simulink model "PI"  (R2024a)
settings: Solver=VariableStepAuto  StartTime=0.0  StopTime=5  RelTol=1e-3
values from neighbouring files (symbols this model uses):
  B = 0    [Parameters.m]
  J = 0.006    [Parameters.m]
  Ls = 0.4    [Parameters.m]
  p = 4    [Parameters.m]
  Rs = 0.02    [Parameters.m]
  samplingTime = 50    [Parameters.m]
  Sm = 0.2205    [Parameters.m]
libraries: slpidlib x3, spsTriangleGeneratorLib x1
settings Model: Creator=anugr  LastModifiedBy=anugr
settings DataIOCC: ReturnWorkspaceOutputs=off

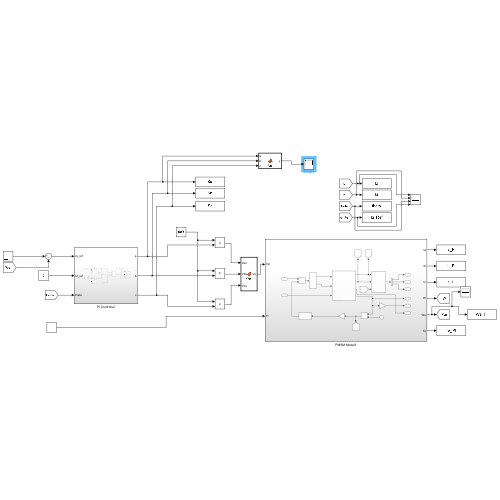
[thumbnail: Simulink's stored preview of the top-level diagram]
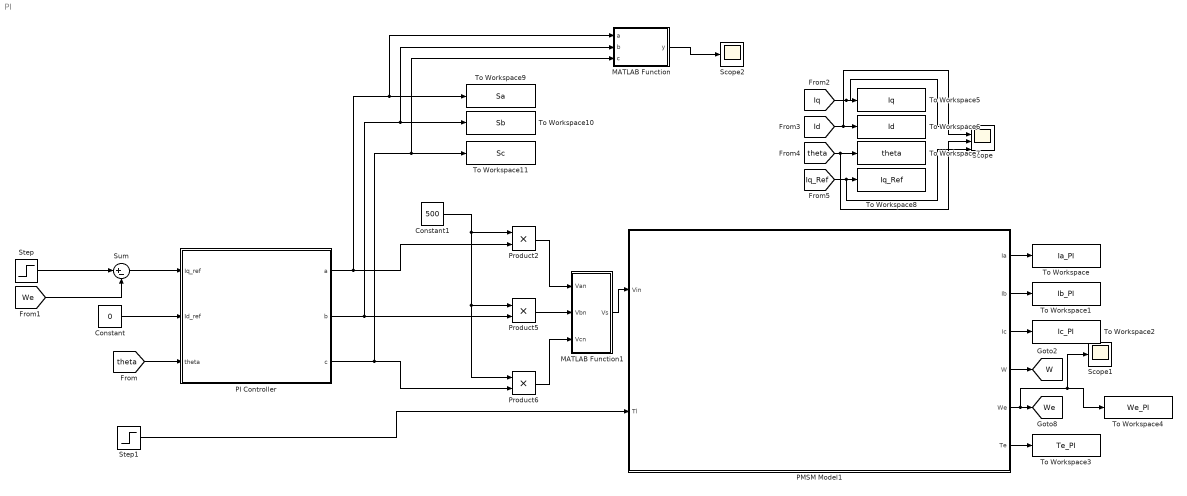
== system PI ==
  Constant : Constant  Value=0
  Constant1 : Constant  Value=500
  MATLAB Function : MATLAB Function  TreatAsAtomicUnit=on
  MATLAB Function1 : MATLAB Function  TreatAsAtomicUnit=on
  PI Controller : Subsystem
  PMSM Model1 : Subsystem
  Product2 : Product
  Product5 : Product
  Product6 : Product
  Scope : Scope  NumInputPorts=4
  Scope1 : Scope
  Scope2 : Scope
  Step : Step  Time=2.5  Before=200  After=400  SampleTime=0
  Step1 : Step  Time=2.5  After=0  SampleTime=0
  Sum : Sum  Inputs=|+-
  To Workspace : ToWorkspace  VariableName=Ia_PI  SaveFormat=Timeseries  SampleTime=-1
  To Workspace1 : ToWorkspace  VariableName=Ib_PI  SaveFormat=Timeseries  SampleTime=-1
  To Workspace10 : ToWorkspace  VariableName=Sb  SampleTime=samplingTime*1e-5
  To Workspace11 : ToWorkspace  VariableName=Sc  SampleTime=samplingTime*1e-5
  To Workspace2 : ToWorkspace  VariableName=Ic_PI  SaveFormat=Timeseries  SampleTime=-1
  To Workspace3 : ToWorkspace  VariableName=Te_PI  SaveFormat=Timeseries  SampleTime=-1
  To Workspace4 : ToWorkspace  VariableName=We_PI  SampleTime=samplingTime * 1e-5
  To Workspace5 : ToWorkspace  VariableName=Iq  SampleTime=samplingTime*1e-5
  To Workspace6 : ToWorkspace  VariableName=Id  SampleTime=samplingTime*1e-5
  To Workspace7 : ToWorkspace  VariableName=theta  SampleTime=samplingTime*1e-5
  To Workspace8 : ToWorkspace  VariableName=Iq_Ref  SampleTime=samplingTime*1e-5
  To Workspace9 : ToWorkspace  VariableName=Sa  SampleTime=samplingTime*1e-5
  tag scope: W=global, We=global
  wires:
  Step/1 -> Sum/1
  Sum/1 -> PI Controller/1(Iq_ref)
  Constant/1 -> PI Controller/2(Id_ref)
  MATLAB Function1/1(Vs) -> PMSM Model1/1(Vin)
  Product5/1 -> MATLAB Function1/2(Vbn)
  PI Controller/1(a) -> MATLAB Function/1(a), To Workspace9/1, Product2/2
  PI Controller/3(c) -> MATLAB Function/3(c), To Workspace11/1, Product6/2
  Constant1/1 -> Product5/1, Product6/1, Product2/1
  PI Controller/2(b) -> MATLAB Function/2(b), To Workspace10/1, Product5/2
  Product6/1 -> MATLAB Function1/3(Vcn)
  Product2/1 -> MATLAB Function1/1(Van)
  PMSM Model1/3(Ic) -> To Workspace2/1
  PMSM Model1/1(Ia) -> To Workspace/1
  PMSM Model1/2(Ib) -> To Workspace1/1
  PMSM Model1/4(W) -> [W]
  PMSM Model1/5(We) -> Scope1/1, To Workspace4/1, [We]
  PMSM Model1/6(Te) -> To Workspace3/1
  Step1/1 -> PMSM Model1/2(Tl)
  [theta] -> PI Controller/3(theta)
  [We] -> Sum/2
  [Iq] -> Scope/1, To Workspace5/1
  [Id] -> Scope/2, To Workspace6/1
  [theta] -> Scope/3, To Workspace7/1
  [Iq_Ref] -> Scope/4, To Workspace8/1
  MATLAB Function/1(y) -> Scope2/1

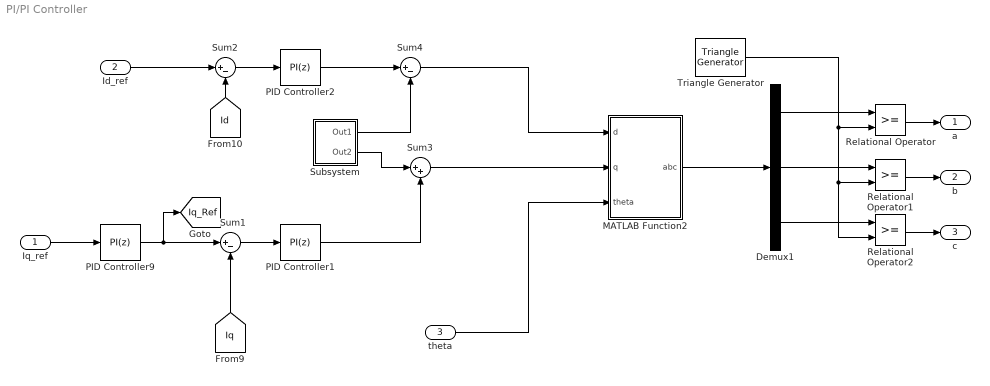
== system PI/PI Controller ==
  Iq_ref : Inport
  Id_ref : Inport  Port=2
  theta : Inport  Port=3
  Demux1 : Demux  Outputs=3
  MATLAB Function2 : MATLAB Function  TreatAsAtomicUnit=on
  PID Controller1 : slpidlib/PID Controller  Controller=PI  Form=Parallel  TimeDomain=Discrete-time  UseExternalTs=off  SampleTime=-1  IntegratorMethod=Forward Euler  FilterMethod=Forward Euler  ControllerParametersSource=internal  P=100  I=30  UseKiTs=off  D=0  UseExternalDerivativeSource=off  N=100  UseFilter=on  TunerSelectOption=Transfer Function Based (PID Tuner App)  InitialConditionSource=internal  InitialConditionForIntegrator=0  InitialConditionForFilter=0  DifferentiatorICPrevScaledInput=0  ExternalReset=none  TrackingMode=off  Kt=1  LimitOutput=off  SatLimitsSource=internal  UpperSaturationLimit=inf  LowerSaturationLimit=-inf  LinearizeAsGain=on  AntiWindupMode=none  Kb=1  LimitIntegrator=off  UpperIntegratorSaturationLimit=inf  LowerIntegratorSaturationLimit=-inf  POutMin=[]  POutMax=[]  IOutMin=[]  IOutMax=[]  DOutMin=[]  DOutMax=[]  NOutMin=[]  NOutMax=[]  SumOutMin=[]  SumOutMax=[]  SaturationOutMin=[]  SaturationOutMax=[]  PParamMin=[]  PParamMax=[]  IParamMin=[]  IParamMax=[]  DParamMin=[]  DParamMax=[]  NParamMin=[]  NParamMax=[]  KbParamMin=[]  KbParamMax=[]  KtParamMin=[]  KtParamMax=[]  KbOutMin=[]  KbOutMax=[]  KtOutMin=[]  KtOutMax=[]  IntegratorOutMin=[]  IntegratorOutMax=[]  FilterOutMin=[]  FilterOutMax=[]  SumI1OutMin=[]  SumI1OutMax=[]  SumI2OutMin=[]  SumI2OutMax=[]  SumI3OutMin=[]  SumI3OutMax=[]  SumI4OutMin=[]  SumI4OutMax=[]  SumDOutMin=[]  SumDOutMax=[]  DifferentiatorOutMin=[]  DifferentiatorOutMax=[]  FilterDiffOutCoefMin=[]  FilterDiffOutCoefMax=[]  ReciprocalOutMin=[]  ReciprocalOutMax=[]  SumDenOutMin=[]  SumDenOutMax=[]  SumNumOutMin=[]  SumNumOutMax=[]  DivideOutMin=[]  DivideOutMax=[]  UdiffTsProdOutMin=[]  UdiffTsProdOutMax=[]  NTsProdOutMin=[]  NTsProdOutMax=[]  UintegralTsProdOutMin=[]  UintegralTsProdOutMax=[]  UngainTsProdOutMin=[]  UngainTsProdOutMax=[]  ClampingZeroOutDataTypeStr=Inherit: Inherit via back propagation  ClampingZeroOutMin=[]  ClampingZeroOutMax=[]  FilterDenConstantOutDataTypeStr=Inherit: Inherit via back propagation  FilterDenConstantOutMin=[]  FilterDenConstantOutMax=[]  PCopyOutDataTypeStr=Inherit: Inherit via back propagation  PCopyOutMin=[]  PCopyOutMax=[]  NCopyOutDataTypeStr=Inherit: Inherit via back propagation  NCopyOutMin=[]  NCopyOutMax=[]  IntegratorContinuousStateAttributes=''  IntegratorStateMustResolveToSignalObject=off  IntegratorRTWStateStorageClass=Auto  FilterContinuousStateAttributes=''  FilterStateMustResolveToSignalObject=off  FilterRTWStateStorageClass=Auto  ParallelPVariant=InternalParameters  IdealPVariant=Disabled  IVariant=InternalParameters  DVariant=Disabled  IntegratorVariant=Discrete  SatVariant=Disabled  AWVariant=Passthrough  PCopyVariant=Disabled  TRVariant=Disabled  FdbkBlocksVariant=Forward  IdealPFdbkVariant=Disabled  SatFdbkVariant=Disabled  DerivativeFilterVariant=Disabled  NVariant=Disabled  NCopyVariant=Disabled_SignalSpec  FilterICVariant=Disabled  IntegratorICVariant=InternalICs  ExternalResetVariant=Disabled  TRSumVariant=Passthrough  SumFdbkVariant=Disabled  SumVariant=Sum_PI  TsampFilterVariant=InternalTs  TsampNgainVariant=Passthrough  TsampIntegralVariant=Disabled_SignalSpec  ExternalSaturationOutDataTypeStr=Inherit: Same as second input  DerivativeSourceVariant=Disabled
  PID Controller2 : slpidlib/PID Controller  Controller=PI  Form=Parallel  TimeDomain=Discrete-time  UseExternalTs=off  SampleTime=-1  IntegratorMethod=Forward Euler  FilterMethod=Forward Euler  ControllerParametersSource=internal  P=100  I=30  UseKiTs=off  D=0  UseExternalDerivativeSource=off  N=100  UseFilter=on  TunerSelectOption=Transfer Function Based (PID Tuner App)  InitialConditionSource=internal  InitialConditionForIntegrator=0  InitialConditionForFilter=0  DifferentiatorICPrevScaledInput=0  ExternalReset=none  TrackingMode=off  Kt=1  LimitOutput=off  SatLimitsSource=internal  UpperSaturationLimit=inf  LowerSaturationLimit=-inf  LinearizeAsGain=on  AntiWindupMode=none  Kb=1  LimitIntegrator=off  UpperIntegratorSaturationLimit=inf  LowerIntegratorSaturationLimit=-inf  POutMin=[]  POutMax=[]  IOutMin=[]  IOutMax=[]  DOutMin=[]  DOutMax=[]  NOutMin=[]  NOutMax=[]  SumOutMin=[]  SumOutMax=[]  SaturationOutMin=[]  SaturationOutMax=[]  PParamMin=[]  PParamMax=[]  IParamMin=[]  IParamMax=[]  DParamMin=[]  DParamMax=[]  NParamMin=[]  NParamMax=[]  KbParamMin=[]  KbParamMax=[]  KtParamMin=[]  KtParamMax=[]  KbOutMin=[]  KbOutMax=[]  KtOutMin=[]  KtOutMax=[]  IntegratorOutMin=[]  IntegratorOutMax=[]  FilterOutMin=[]  FilterOutMax=[]  SumI1OutMin=[]  SumI1OutMax=[]  SumI2OutMin=[]  SumI2OutMax=[]  SumI3OutMin=[]  SumI3OutMax=[]  SumI4OutMin=[]  SumI4OutMax=[]  SumDOutMin=[]  SumDOutMax=[]  DifferentiatorOutMin=[]  DifferentiatorOutMax=[]  FilterDiffOutCoefMin=[]  FilterDiffOutCoefMax=[]  ReciprocalOutMin=[]  ReciprocalOutMax=[]  SumDenOutMin=[]  SumDenOutMax=[]  SumNumOutMin=[]  SumNumOutMax=[]  DivideOutMin=[]  DivideOutMax=[]  UdiffTsProdOutMin=[]  UdiffTsProdOutMax=[]  NTsProdOutMin=[]  NTsProdOutMax=[]  UintegralTsProdOutMin=[]  UintegralTsProdOutMax=[]  UngainTsProdOutMin=[]  UngainTsProdOutMax=[]  ClampingZeroOutDataTypeStr=Inherit: Inherit via back propagation  ClampingZeroOutMin=[]  ClampingZeroOutMax=[]  FilterDenConstantOutDataTypeStr=Inherit: Inherit via back propagation  FilterDenConstantOutMin=[]  FilterDenConstantOutMax=[]  PCopyOutDataTypeStr=Inherit: Inherit via back propagation  PCopyOutMin=[]  PCopyOutMax=[]  NCopyOutDataTypeStr=Inherit: Inherit via back propagation  NCopyOutMin=[]  NCopyOutMax=[]  IntegratorContinuousStateAttributes=''  IntegratorStateMustResolveToSignalObject=off  IntegratorRTWStateStorageClass=Auto  FilterContinuousStateAttributes=''  FilterStateMustResolveToSignalObject=off  FilterRTWStateStorageClass=Auto  ParallelPVariant=InternalParameters  IdealPVariant=Disabled  IVariant=InternalParameters  DVariant=Disabled  IntegratorVariant=Discrete  SatVariant=Disabled  AWVariant=Passthrough  PCopyVariant=Disabled  TRVariant=Disabled  FdbkBlocksVariant=Forward  IdealPFdbkVariant=Disabled  SatFdbkVariant=Disabled  DerivativeFilterVariant=Disabled  NVariant=Disabled  NCopyVariant=Disabled_SignalSpec  FilterICVariant=Disabled  IntegratorICVariant=InternalICs  ExternalResetVariant=Disabled  TRSumVariant=Passthrough  SumFdbkVariant=Disabled  SumVariant=Sum_PI  TsampFilterVariant=InternalTs  TsampNgainVariant=Passthrough  TsampIntegralVariant=Disabled_SignalSpec  ExternalSaturationOutDataTypeStr=Inherit: Same as second input  DerivativeSourceVariant=Disabled
  PID Controller9 : slpidlib/PID Controller  Controller=PI  Form=Parallel  TimeDomain=Discrete-time  UseExternalTs=off  SampleTime=-1  IntegratorMethod=Forward Euler  FilterMethod=Forward Euler  ControllerParametersSource=internal  P=0.1  I=1  UseKiTs=off  D=0  UseExternalDerivativeSource=off  N=100  UseFilter=on  TunerSelectOption=Transfer Function Based (PID Tuner App)  InitialConditionSource=internal  InitialConditionForIntegrator=0  InitialConditionForFilter=0  DifferentiatorICPrevScaledInput=0  ExternalReset=none  TrackingMode=off  Kt=1  LimitOutput=off  SatLimitsSource=internal  UpperSaturationLimit=inf  LowerSaturationLimit=-inf  LinearizeAsGain=on  AntiWindupMode=none  Kb=1  LimitIntegrator=off  UpperIntegratorSaturationLimit=inf  LowerIntegratorSaturationLimit=-inf  POutMin=[]  POutMax=[]  IOutMin=[]  IOutMax=[]  DOutMin=[]  DOutMax=[]  NOutMin=[]  NOutMax=[]  SumOutMin=[]  SumOutMax=[]  SaturationOutMin=[]  SaturationOutMax=[]  PParamMin=[]  PParamMax=[]  IParamMin=[]  IParamMax=[]  DParamMin=[]  DParamMax=[]  NParamMin=[]  NParamMax=[]  KbParamMin=[]  KbParamMax=[]  KtParamMin=[]  KtParamMax=[]  KbOutMin=[]  KbOutMax=[]  KtOutMin=[]  KtOutMax=[]  IntegratorOutMin=[]  IntegratorOutMax=[]  FilterOutMin=[]  FilterOutMax=[]  SumI1OutMin=[]  SumI1OutMax=[]  SumI2OutMin=[]  SumI2OutMax=[]  SumI3OutMin=[]  SumI3OutMax=[]  SumI4OutMin=[]  SumI4OutMax=[]  SumDOutMin=[]  SumDOutMax=[]  DifferentiatorOutMin=[]  DifferentiatorOutMax=[]  FilterDiffOutCoefMin=[]  FilterDiffOutCoefMax=[]  ReciprocalOutMin=[]  ReciprocalOutMax=[]  SumDenOutMin=[]  SumDenOutMax=[]  SumNumOutMin=[]  SumNumOutMax=[]  DivideOutMin=[]  DivideOutMax=[]  UdiffTsProdOutMin=[]  UdiffTsProdOutMax=[]  NTsProdOutMin=[]  NTsProdOutMax=[]  UintegralTsProdOutMin=[]  UintegralTsProdOutMax=[]  UngainTsProdOutMin=[]  UngainTsProdOutMax=[]  ClampingZeroOutDataTypeStr=Inherit: Inherit via back propagation  ClampingZeroOutMin=[]  ClampingZeroOutMax=[]  FilterDenConstantOutDataTypeStr=Inherit: Inherit via back propagation  FilterDenConstantOutMin=[]  FilterDenConstantOutMax=[]  PCopyOutDataTypeStr=Inherit: Inherit via back propagation  PCopyOutMin=[]  PCopyOutMax=[]  NCopyOutDataTypeStr=Inherit: Inherit via back propagation  NCopyOutMin=[]  NCopyOutMax=[]  IntegratorContinuousStateAttributes=''  IntegratorStateMustResolveToSignalObject=off  IntegratorRTWStateStorageClass=Auto  FilterContinuousStateAttributes=''  FilterStateMustResolveToSignalObject=off  FilterRTWStateStorageClass=Auto  ParallelPVariant=InternalParameters  IdealPVariant=Disabled  IVariant=InternalParameters  DVariant=Disabled  IntegratorVariant=Discrete  SatVariant=Disabled  AWVariant=Passthrough  PCopyVariant=Disabled  TRVariant=Disabled  FdbkBlocksVariant=Forward  IdealPFdbkVariant=Disabled  SatFdbkVariant=Disabled  DerivativeFilterVariant=Disabled  NVariant=Disabled  NCopyVariant=Disabled_SignalSpec  FilterICVariant=Disabled  IntegratorICVariant=InternalICs  ExternalResetVariant=Disabled  TRSumVariant=Passthrough  SumFdbkVariant=Disabled  SumVariant=Sum_PI  TsampFilterVariant=InternalTs  TsampNgainVariant=Passthrough  TsampIntegralVariant=Disabled_SignalSpec  ExternalSaturationOutDataTypeStr=Inherit: Same as second input  DerivativeSourceVariant=Disabled
  Relational Operator : RelationalOperator  OutDataTypeStr=boolean  RndMeth=Simplest  InputSameDT=off
  Relational Operator1 : RelationalOperator  OutDataTypeStr=boolean  RndMeth=Simplest  InputSameDT=off
  Relational Operator2 : RelationalOperator  OutDataTypeStr=boolean  RndMeth=Simplest  InputSameDT=off
  Subsystem : Subsystem
  Sum1 : Sum  Inputs=|+-
  Sum2 : Sum  Inputs=|+-
  Sum3 : Sum  Inputs=|++
  Sum4 : Sum  Inputs=|+-
  Triangle Generator : spsTriangleGeneratorLib/Triangle Generator  Freq=1e3  Phase=90  Ts=0
  a : Outport
  b : Outport  Port=2
  c : Outport  Port=3
  tag scope: Iq_Ref=global
  wires:
  Demux1/2 -> Relational Operator1/1
  PID Controller9/1 -> [Iq_Ref], Sum1/1
  Sum2/1 -> PID Controller2/1
  Demux1/3 -> Relational Operator2/1
  Subsystem/1(Out1) -> Sum4/2
  MATLAB Function2/1(abc) -> Demux1/1
  Relational Operator2/1 -> c/1
  [Id] -> Sum2/2
  PID Controller1/1 -> Sum3/2
  Triangle Generator/1 -> Relational Operator2/2, Relational Operator1/2, Relational Operator/2
  Subsystem/2(Out2) -> Sum3/1
  Demux1/1 -> Relational Operator/1
  theta/1 -> MATLAB Function2/3(theta)
  PID Controller2/1 -> Sum4/1
  Sum4/1 -> MATLAB Function2/1(d)
  Id_ref/1 -> Sum2/1
  Iq_ref/1 -> PID Controller9/1
  Sum3/1 -> MATLAB Function2/2(q)
  Sum1/1 -> PID Controller1/1
  [Iq] -> Sum1/2
  Relational Operator1/1 -> b/1
  Relational Operator/1 -> a/1

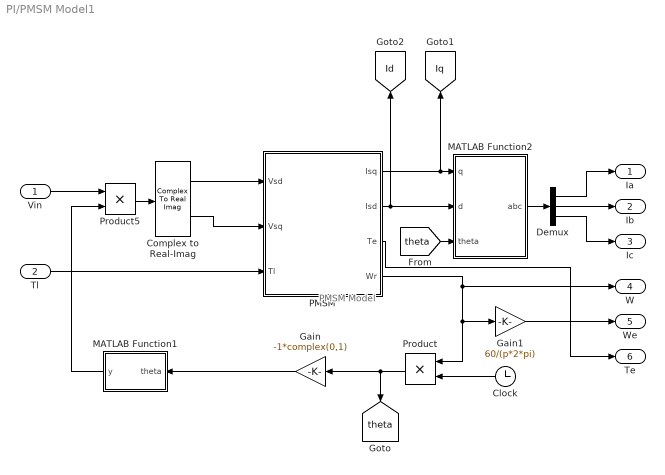
== system PI/PMSM Model1 ==
  note: PMSM Model
  Vin : Inport
  Tl : Inport  Port=2
  Clock : Clock
  Complex to Real-Imag : ComplexToRealImag
  Demux : Demux  Outputs=3
  Gain : Gain  Gain=-1*complex(0,1)
  Gain1 : Gain  Gain=60/(p*2*pi)
  MATLAB Function1 : MATLAB Function  TreatAsAtomicUnit=on
  MATLAB Function2 : MATLAB Function  TreatAsAtomicUnit=on
  PMSM : Subsystem
  Product : Product
  Product5 : Product
  Ia : Outport
  Ib : Outport  Port=2
  Ic : Outport  Port=3
  W : Outport  Port=4
  We : Outport  Port=5
  Te : Outport  Port=6
  tag scope: Id=global, Iq=global, theta=global
  wires:
  Tl/1 -> PMSM/3(Tl)
  PMSM/4(Wr) -> W/1, Gain1/1, Product/1
  Product/1 -> Gain/1, [theta]
  Demux/3 -> Ic/1
  Clock/1 -> Product/2
  PMSM/1(Isq) -> [Iq], MATLAB Function2/1(q)
  MATLAB Function1/1(y) -> Product5/2
  Complex to Real-Imag/1 -> PMSM/1(Vsd)
  PMSM/3(Te) -> Te/1
  PMSM/2(Isd) -> MATLAB Function2/2(d), [Id]
  Complex to Real-Imag/2 -> PMSM/2(Vsq)
  Product5/1 -> Complex to Real-Imag/1
  Gain/1 -> MATLAB Function1/1(theta)
  Demux/1 -> Ia/1
  MATLAB Function2/1(abc) -> Demux/1
  Vin/1 -> Product5/1
  Gain1/1 -> We/1
  Demux/2 -> Ib/1
  [theta] -> MATLAB Function2/3(theta)

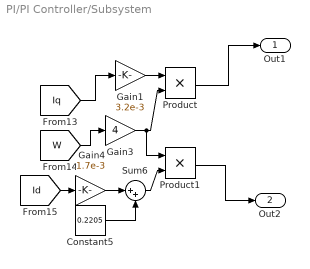
== system PI/PI Controller/Subsystem ==
  Constant5 : Constant  Value=0.2205
  Gain1 : Gain  Gain=3.2e-3
  Gain3 : Gain  Gain=4
  Gain4 : Gain  Gain=1.7e-3
  Product : Product
  Product1 : Product
  Sum6 : Sum  Inputs=|++
  Out1 : Outport
  Out2 : Outport  Port=2
  wires:
  [W] -> Gain3/1
  [Id] -> Gain4/1
  [Iq] -> Gain1/1
  Gain4/1 -> Sum6/1
  Gain1/1 -> Product/1
  Sum6/1 -> Product1/2
  Gain3/1 -> Product1/1, Product/2
  Constant5/1 -> Sum6/2
  Product/1 -> Out1/1
  Product1/1 -> Out2/1

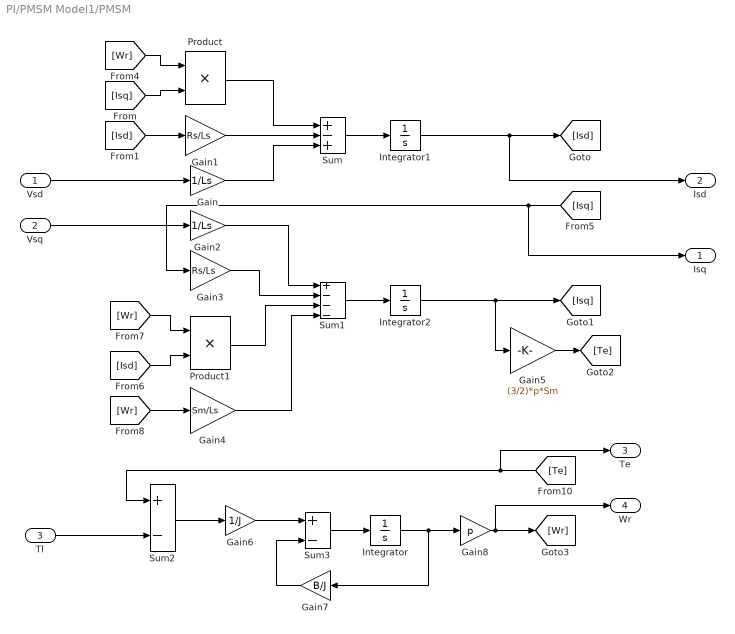
== system PI/PMSM Model1/PMSM ==
  Vsd : Inport
  Vsq : Inport  Port=2
  Tl : Inport  Port=3
  Gain : Gain  Gain=1/Ls
  Gain1 : Gain  Gain=Rs/Ls
  Gain2 : Gain  Gain=1/Ls
  Gain3 : Gain  Gain=Rs/Ls
  Gain4 : Gain  Gain=Sm/Ls
  Gain5 : Gain  Gain=(3/2)*p*Sm
  Gain6 : Gain  Gain=1/J
  Gain7 : Gain  Gain=B/J
  Gain8 : Gain  Gain=p
  Integrator : Integrator
  Integrator1 : Integrator
  Integrator2 : Integrator
  Product : Product
  Product1 : Product
  Sum : Sum  Inputs=+-+
  Sum1 : Sum  Inputs=+---
  Sum2 : Sum  Inputs=+-
  Sum3 : Sum  Inputs=+-
  Isq : Outport
  Isd : Outport  Port=2
  Te : Outport  Port=3
  Wr : Outport  Port=4
  wires:
  Gain5/1 -> [Te]
  [Wr] -> Gain4/1
  [Isq] -> Isq/1, Gain3/1
  [Te] -> Te/1, Sum2/1
  Integrator2/1 -> Gain5/1, [Isq]
  Gain6/1 -> Sum3/1
  Sum1/1 -> Integrator2/1
  Gain/1 -> Sum/3
  Integrator/1 -> Gain8/1, Gain7/1
  Tl/1 -> Sum2/2
  Gain8/1 -> Wr/1, [Wr]
  Gain2/1 -> Sum1/1
  Sum3/1 -> Integrator/1
  Vsd/1 -> Gain/1
  Sum2/1 -> Gain6/1
  [Isd] -> Product1/2
  Gain7/1 -> Sum3/2
  Gain3/1 -> Sum1/2
  Gain4/1 -> Sum1/4
  [Wr] -> Product/1
  [Isq] -> Product/2
  Product1/1 -> Sum1/3
  [Wr] -> Product1/1
  Product/1 -> Sum/1
  Gain1/1 -> Sum/2
  [Isd] -> Gain1/1
  Sum/1 -> Integrator1/1
  Vsq/1 -> Gain2/1
  Integrator1/1 -> Isd/1, [Isd]

== matlab function PI/MATLAB Function ==
  data: a input; y output; b input; c input
function y = fcn(a, b, c)

y = 4*a + 2*b + c;

== matlab function PI/MATLAB Function1 ==
  data: Van input; Vs output; Vbn input; Vcn input
function Vs = fcn(Van,Vbn,Vcn)

a=complex(cos(2*pi/3),sin(2*pi/3)); 
Vs =(2/3)*(Van+(a*Vbn)+((a^2)*Vcn)) ;

== matlab function PI/PMSM Model1/MATLAB Function1 ==
  data: theta input; y output
function y = fcn(theta)

y = exp((theta));

== matlab function PI/PMSM Model1/MATLAB Function2 ==
  data: q input; d input; abc output; theta input
function abc = dq_to_abc(q, d, theta)
    % Inputs:
    % d, q   : DQ components
    % theta  : Electrical angle in radians

    % Transformation matrix
    T = [cos(theta), -sin(theta), 1; 
         cos(theta - 2*pi/3), -sin(theta - 2*pi/3), 1; 
         cos(theta + 2*pi/3), -sin(theta + 2*pi/3), 1];

    % Calculate abc components
    abc = (2/3) * T * [d; q; 0];
end

== matlab function PI/PI Controller/MATLAB Function2 ==
  data: d input; q input; abc output; theta input
function abc = dq_to_abc(d, q, theta)
    % Inputs:
    % d, q   : DQ components
    % theta  : Electrical angle in radians

    % Transformation matrix
    T = [cos(theta), -sin(theta), 1; 
         cos(theta - 2*pi/3), -sin(theta - 2*pi/3), 1; 
         cos(theta + 2*pi/3), -sin(theta + 2*pi/3), 1];

    % Calculate abc components
    abc = (2/3) * T * [d; q; 0];
end
